simulink model "bola_saltitonaP31"  (R2015a)
settings: Solver=ode3  StartTime=0.0  StopTime=13  FixedStep=1e-4  RelTol=1e-3
libraries: simulink x2
settings Model: Creator=ModSim  LastModifiedBy=João Santos
settings DataIOCC: InspectSignalLogs=on
settings DebuggingCC: MaxConsecutiveZCsMsg=none

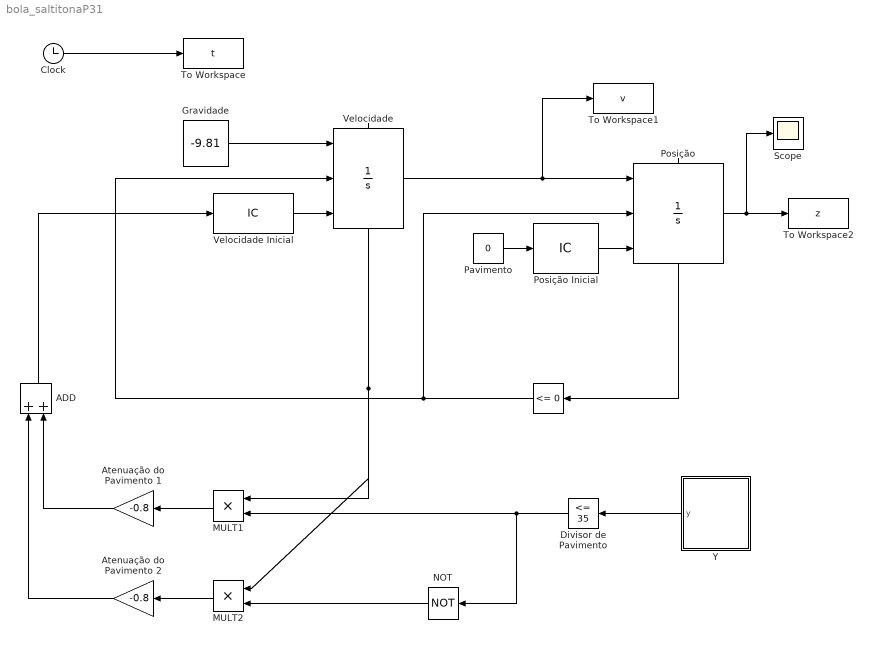
== system bola_saltitonaP31 ==
  " " : simulink/Logic and Bit Operations/Compare To Zero  relop=<=  OutDataTypeStr=boolean
  " Posição" : Integrator  ExternalReset=rising  InitialConditionSource=external  LimitOutput=on  LowerSaturationLimit=0  ShowStatePort=on
  " Atenuação do Pavimento 2" : Gain  Gain=-0.8
  ADD : Sum
  Atenuação do Pavimento 1 : Gain  Gain=-0.8
  Clock : Clock
      settings: Decimation=100
  Divisor de Pavimento : simulink/Logic and Bit Operations/Compare To Constant  relop=<=  const=35  OutDataTypeStr=boolean
  Gravidade : Constant  Value=-9.81
  MULT1 : Product
  "MULT2 " : Product
  NOT : Logic  Operator=NOT  IconShape=distinctive  AllPortsSameDT=off  OutDataTypeStr=boolean
  Pavimento : Constant  Value=0
  Posição Inicial : InitialCondition  Value=10
  Scope : Scope
  To Workspace : ToWorkspace  VariableName=t  SampleTime=-1
  To Workspace1 : ToWorkspace  VariableName=v  SampleTime=-1
  To Workspace2 : ToWorkspace  VariableName=z  SampleTime=-1
  Velocidade : Integrator  ExternalReset=rising  InitialConditionSource=external  ShowStatePort=on
  Velocidade Inicial : InitialCondition  Value=0
  Y : Subsystem
  wires:
  Velocidade Inicial/1 -> Velocidade/3
  " "/1 -> Velocidade/2, " Posição"/2
  Clock/1 -> To Workspace/1
  Posição Inicial/1 -> " Posição"/3
  Pavimento/1 -> Posição Inicial/1
  " Posição"/1 -> To Workspace2/1, Scope/1
  Velocidade/1 -> " Posição"/1, To Workspace1/1
  Gravidade/1 -> Velocidade/1
  " Posição"/State -> " "/1
  Atenuação do Pavimento 1/1 -> ADD/2
  " Atenuação do Pavimento 2"/1 -> ADD/1
  ADD/1 -> Velocidade Inicial/1
  MULT1/1 -> Atenuação do Pavimento 1/1
  "MULT2 "/1 -> " Atenuação do Pavimento 2"/1
  Divisor de Pavimento/1 -> MULT1/2, NOT/1
  NOT/1 -> "MULT2 "/2
  Velocidade/State -> "MULT2 "/1, MULT1/1
  Y/1(y) -> Divisor de Pavimento/1

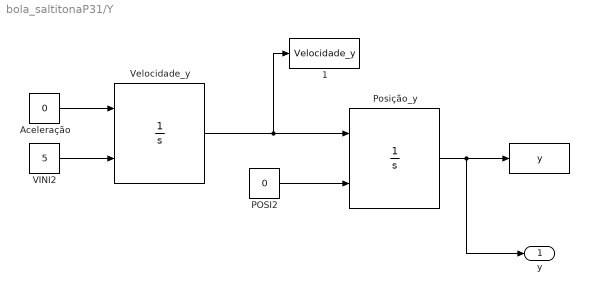
== system bola_saltitonaP31/Y ==
  " Posição_y" : Integrator  InitialConditionSource=external  LimitOutput=on  LowerSaturationLimit=0
  " " : ToWorkspace  VariableName=y  SampleTime=-1
  " 1" : ToWorkspace  VariableName=Velocidade_y  SampleTime=-1
  Aceleração : Constant  Value=0
  POSI2 : Constant  Value=0
  VINI2 : Constant  Value=5
  Velocidade_y : Integrator  InitialConditionSource=external  LowerSaturationLimit=0
  y : Outport
  wires:
  " Posição_y"/1 -> y/1, " "/1
  Velocidade_y/1 -> " 1"/1, " Posição_y"/1
  POSI2/1 -> " Posição_y"/2
  Aceleração/1 -> Velocidade_y/1
  VINI2/1 -> Velocidade_y/2
